simulink model "HIL_model_overall"  (R2014a)
settings: Solver=ode5  StartTime=0.0  StopTime=simulationTime  FixedStep=0.1  RelTol=1e-3
values from neighbouring files (symbols this model uses):
  A_ref = [0.176     0           0 ... (first row only)    [theProgram.m]
  B_ref = [0.0554     0           0 ... (first row only)    [theProgram.m]
  C_ref = [0.05*0.0038     0           0 ... (first row only)    [theProgram.m]
  Di = [50 0 ... (first row only)    [theProgram.m]
  Dist_spv_rfp = sqrt( ( shipL_d(1) - Rfp(1) )^2 + (shipL_d(2) - Rfp(2) )^2 )    [theProgram.m]
  Ds = [-X_u 0 0 ... (first row only)    [theProgram.m]
  iceDiameter = 0.2    [theProgram.m]
  K2_obs = diag([0.25 1 0.5])    [theProgram.m]
  K3_obs = diag([1 1 1])    [theProgram.m]
  K4_obs = diag([250 300 100])    [theProgram.m]
  K_M = [ 1 0 0 ... (first row only)    [theProgram.m]
  K_tow = 20    [theProgram.m]
  kappa = 2    [theProgram.m]
  Kd = [50 0 0 ... (first row only)    [theProgram.m]
  Kp = [10 0 0 ... (first row only)    [theProgram.m]
  Mi_a = iceMass*[1 0; 0 1]    [theProgram.m]
  Mi_rb = iceMass*[1 0; 0 1]    [theProgram.m]
  Ms_a = -[X_udot 0 0 ... (first row only)    [theProgram.m]
  Ms_rb = [shipMass 0 0 ... (first row only)    [theProgram.m]
  Ms_tot = Ms_rb + Ms_a    [theProgram.m]
  Ninstances = 50    [theProgram.m]
  nPoints = size(WP,1)    [theProgram.m]
  Offset_direction = 0    [theProgram.m]
  overturnLimit = 4    [theProgram.m]
  Piceberg = [-4.5; -2.9]    [theProgram.m]
  Pship = [-3.5; -2.9; 0]    [theProgram.m]
  ruptureLimit = 3    [theProgram.m]
  ruptureLimitRef = 9    [theProgram.m]
  ruptureNear = 9.5    [theProgram.m]
  S_trans = [0 -1 0 ... (first row only)    [theProgram.m]
  saved_init = zeros(Ninstances,1)    [theProgram.m]
  sd_break = 0.075*T_break    (= 12)    [theProgram.m]
  sd_overturn = 0.075*T_overturn    (= 9.75)    [theProgram.m]
  sd_slip = 0.075*T_slip    (= 10.5)    [theProgram.m]
  shipL_d = [shipLength-0.55; 0]    [theProgram.m]
  sigma = 0.005    [theProgram.m]
  slippageLimit = 5    [theProgram.m]
  T_bias = diag([20 200 20])    [theProgram.m]
  T_break = 160    [theProgram.m]
  T_overturn = 130    [theProgram.m]
  T_slip = 140    [theProgram.m]
  TowLineLength = 1.11    [theProgram.m]
  u_ref = 0.03    [theProgram.m]
  u_surge_max = 2    [theProgram.m]
  u_sway_max = 1    [theProgram.m]
  u_yaw_max = 2*pi/60    (= 0.10471975512)    [theProgram.m]
  Vc = [cVelocity*cos(cAngle) ... (first row only)    [theProgram.m]
  WP = [-5 -3 ... (first row only)    [theProgram.m]
  WPi_init = 2    [theProgram.m]
libraries: dspmtrx3 x2
(part 1 of 2)
settings Model: Creator=Andreas  LastModifiedBy=mclab
settings DebuggingCC: UnderspecifiedInitializationDetection=Classic  StateNameClashWarn=warning

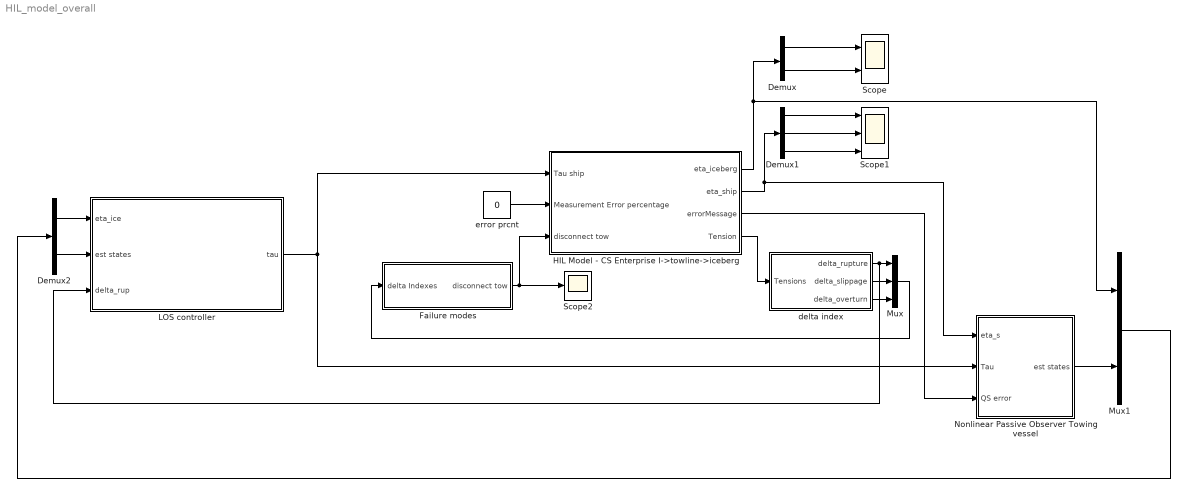
== system HIL_model_overall ==
  Demux : Demux  Outputs=2
  Demux1 : Demux  Outputs=3
  Demux2 : Demux  Outputs=[2; 9]
  Failure modes : Subsystem
  HIL Model - CS Enterprise I->towline->iceberg : Subsystem  VariantControl=Variant1
  LOS controller : Subsystem
  Mux : Mux  Inputs=3
  Mux1 : Mux  Inputs=[2; 9]
  Nonlinear Passive Observer Towing vessel : Subsystem
  Scope : Scope  NumInputPorts=2
      settings: YMin=-5~-5  YMax=5~5  SaveName=ScopeData5
  Scope1 : Scope  NumInputPorts=3
      settings: YMin=-5~-5~-5  YMax=5~5~5  SaveName=ScopeData6
  Scope2 : Scope
      settings: SaveName=ScopeData7
  delta index : Subsystem
  error prcnt : Constant  Value=0
  wires:
  error prcnt/1 -> HIL Model - CS Enterprise I->towline->iceberg/2(Measurement Error percentage)
  HIL Model - CS Enterprise I->towline->iceberg/4(Tension) -> delta index/1(Tensions)
  Failure modes/1(disconnect tow) -> HIL Model - CS Enterprise I->towline->iceberg/3(disconnect tow), Scope2/1
  delta index/2(delta_slippage) -> Mux/2
  delta index/3(delta_overturn) -> Mux/3
  delta index/1(delta_rupture) -> LOS controller/3(delta_rup), Mux/1
  Mux/1 -> Failure modes/1(delta Indexes)
  LOS controller/1(tau) -> HIL Model - CS Enterprise I->towline->iceberg/1(Tau ship), Nonlinear Passive Observer Towing vessel/2(Tau)
  HIL Model - CS Enterprise I->towline->iceberg/1(eta_iceberg) -> Mux1/1, Demux/1
  Demux/2 -> Scope/2
  Demux/1 -> Scope/1
  HIL Model - CS Enterprise I->towline->iceberg/2(eta_ship) -> Nonlinear Passive Observer Towing vessel/1(eta_s), Demux1/1
  Demux1/2 -> Scope1/2
  Demux1/3 -> Scope1/3
  Demux1/1 -> Scope1/1
  HIL Model - CS Enterprise I->towline->iceberg/3(errorMessage) -> Nonlinear Passive Observer Towing vessel/3(QS error)
  Nonlinear Passive Observer Towing vessel/1(est states) -> Mux1/2
  Demux2/2 -> LOS controller/2(est states)
  Demux2/1 -> LOS controller/1(eta_ice)
  Mux1/1 -> Demux2/1

== system HIL_model_overall/Failure modes ==
  delta Indexes : Inport
  Clock : Clock
  MATLAB Function : MATLAB Function  TreatAsAtomicUnit=on
  Memory : Memory
  To Workspace : ToWorkspace  VariableName=isDisconnected  SaveFormat=Timeseries  SampleTime=-1
  limits : Constant  Value=[overturnLimit; ruptureLimit; slippageLimit]  VectorParams1D=off
  disconnect tow : Outport
  wires:
  limits/1 -> MATLAB Function/2(limits)
  delta Indexes/1 -> MATLAB Function/1(deltaIndex)
  Clock/1 -> MATLAB Function/4(theTime)
  MATLAB Function/1(disconnect) -> Memory/1
  Memory/1 -> To Workspace/1, MATLAB Function/3(preDisconnect), disconnect tow/1

== system HIL_model_overall/HIL Model - CS Enterprise I->towline->iceberg ==
  Tau ship : Inport
  Measurement Error percentage : Inport  Port=2
  disconnect tow : Inport  Port=3
  Demux : Demux  Outputs=2
  Mux : Mux  Inputs=[3; 2]
  Ship - Iceberg - Current Model : Subsystem
  Tension estimator : Subsystem
  eta_iceberg : Outport
  eta_ship : Outport  Port=2
  errorMessage : Outport  Port=3
  Tension : Outport  Port=4
  wires:
  Tension estimator/2(T_2dof iceberg) -> Ship - Iceberg - Current Model/2(Tension 2D)
  Tension estimator/1(T_3dof ship) -> Ship - Iceberg - Current Model/1(Tension 3D)
  Measurement Error percentage/1 -> Ship - Iceberg - Current Model/4(error percentage)
  Demux/2 -> Tension estimator/2(eta_i)
  Ship - Iceberg - Current Model/1(eta_i) -> Mux/2, eta_iceberg/1
  Demux/1 -> Tension estimator/1(eta_s)
  Tau ship/1 -> Ship - Iceberg - Current Model/3(tau ship)
  Ship - Iceberg - Current Model/3(error) -> errorMessage/1
  Mux/1 -> Demux/1
  Ship - Iceberg - Current Model/2(eta_s) -> Mux/1, eta_ship/1
  Tension estimator/3(Tension) -> Tension/1
  disconnect tow/1 -> Tension estimator/3(Disconnect towline)

== system HIL_model_overall/LOS controller ==
  eta_ice : Inport
  est states : Inport  Port=2
  delta_rup : Inport  Port=3
  Demux : Demux  Outputs=[3; 3; 3]
  LOS iceberg : Subsystem
  "Point Controller,  backstepping" : Subsystem
  Reference Model : Subsystem
  Waypoints : Constant  Value=WP  VectorParams1D=off
  tau : Outport
  wires:
  eta_ice/1 -> Reference Model/1(eta_ice), LOS iceberg/1(eta_ice)
  Demux/1 -> Reference Model/6(eta_ship est), "Point Controller,  backstepping"/4(eta_s est)
  Demux/2 -> Reference Model/7(nu_ship est), "Point Controller,  backstepping"/5(nu_s est)
  "Point Controller,  backstepping"/1(tau) -> tau/1
  Waypoints/1 -> LOS iceberg/2(WP), Reference Model/5(WP)
  est states/1 -> Demux/1
  Demux/3 -> "Point Controller,  backstepping"/6(b_s est)
  Reference Model/1(eta_d) -> "Point Controller,  backstepping"/1(eta_d)
  Reference Model/2(nu_d) -> "Point Controller,  backstepping"/2(nu_d)
  Reference Model/3(nu_dot_d) -> "Point Controller,  backstepping"/3(nu_dot_d)
  LOS iceberg/1(alpha_iceberg) -> Reference Model/2(alpha_LOS)
  LOS iceberg/2(WPi) -> Reference Model/3(WPi)
  LOS iceberg/3(alphaIce_save) -> Reference Model/4(alpha_LOS_saved)
  delta_rup/1 -> Reference Model/8(delta_rup)

== system HIL_model_overall/Nonlinear Passive Observer Towing vessel ==
  eta_s : Inport
  Tau : Inport  Port=2
  QS error : Inport  Port=3
  Mux : Mux  Inputs=[3; 3; 3]
  To Workspace : ToWorkspace  VariableName=QSerror  SaveFormat=Timeseries  SampleTime=-1
  estimation : Subsystem
  est states : Outport
  wires:
  eta_s/1 -> estimation/1(eta_s)
  estimation/1(eta_s est) -> Mux/1
  Tau/1 -> estimation/2(Tau)
  estimation/2(nu_s est) -> Mux/2
  estimation/3(b_s est) -> Mux/3
  Mux/1 -> est states/1
  QS error/1 -> To Workspace/1, estimation/3(QS error)

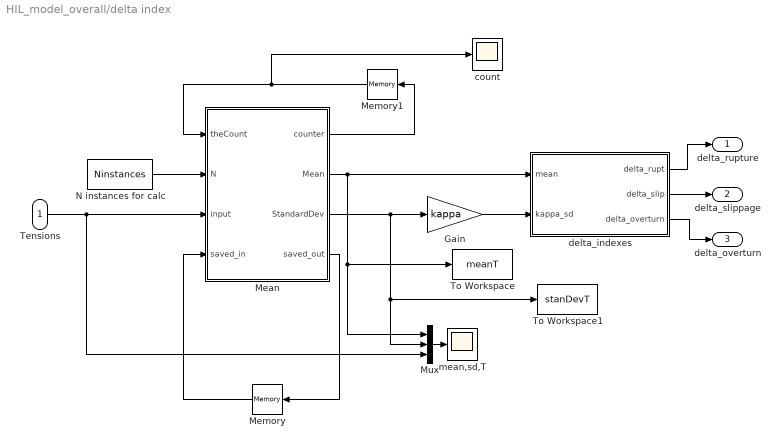
== system HIL_model_overall/delta index ==
  Tensions : Inport
  Gain : Gain  Gain=kappa
  Mean : MATLAB Function  TreatAsAtomicUnit=on
  Memory : Memory  X0=saved_init
  Memory1 : Memory  X0=1
  Mux : Mux  Inputs=3
  N instances for calc : Constant  Value=Ninstances
  To Workspace : ToWorkspace  VariableName=meanT  SaveFormat=Timeseries  SampleTime=-1
  To Workspace1 : ToWorkspace  VariableName=stanDevT  SaveFormat=Timeseries  SampleTime=-1
  count : Scope
  delta_indexes : Subsystem
  mean,sd,T : Scope
      settings: SaveName=ScopeData2
  delta_rupture : Outport
  delta_slippage : Outport  Port=2
  delta_overturn : Outport  Port=3
  wires:
  Mux/1 -> mean,sd,T/1
  Memory/1 -> Mean/4(saved_in)
  Memory1/1 -> Mean/1(theCount), count/1
  Mean/3(StandardDev) -> To Workspace1/1, Mux/2, Gain/1
  Mean/1(counter) -> Memory1/1
  N instances for calc/1 -> Mean/2(N)
  Mean/4(saved_out) -> Memory/1
  Mean/2(Mean) -> To Workspace/1, Mux/1, delta_indexes/1(mean)
  Tensions/1 -> Mux/3, Mean/3(input)
  Gain/1 -> delta_indexes/2(kappa_sd)
  delta_indexes/1(delta_rupt) -> delta_rupture/1
  delta_indexes/2(delta_slip) -> delta_slippage/1
  delta_indexes/3(delta_overturn) -> delta_overturn/1

== system HIL_model_overall/HIL Model - CS Enterprise I->towline->iceberg/Ship - Iceberg - Current Model ==
  Tension 3D : Inport
  Tension 2D : Inport  Port=2
  tau ship : Inport  Port=3
  error percentage : Inport  Port=4
  Current model : Subsystem
  Iceberg model : Subsystem
  MC Lab Signal Fault : MATLAB Function  TreatAsAtomicUnit=on
  Memory : Memory  X0=[0; 0]
  Memory1 : Memory  X0=[0; 0; 0]
  Memory2 : Memory
  Ship model : Subsystem
  eta_i : Outport
  eta_s : Outport  Port=2
  error : Outport  Port=3
  wires:
  Memory2/1 -> MC Lab Signal Fault/4(error_previous)
  Memory1/1 -> MC Lab Signal Fault/5(eta_s_previous)
  Memory/1 -> MC Lab Signal Fault/6(eta_i_previous)
  MC Lab Signal Fault/1(error) -> error/1, Memory2/1
  MC Lab Signal Fault/3(eta_i) -> eta_i/1, Memory/1
  MC Lab Signal Fault/2(eta_s) -> eta_s/1, Memory1/1
  Iceberg model/1(eta_i) -> MC Lab Signal Fault/3(eta_i_in)
  Ship model/2(eta_s) -> MC Lab Signal Fault/2(eta_s_in)
  error percentage/1 -> MC Lab Signal Fault/1(err_percent)
  Ship model/3(nu_s) -> Current model/2(nu_s)  "nu_s"
  Ship model/1(R(psi)^T) -> Current model/1(R(psi) transposed)
  Tension 2D/1 -> Iceberg model/3(T)
  Current model/4(Vc_dot) -> Iceberg model/2(Vc_dot)
  Current model/3(Vc) -> Iceberg model/1(Vc)
  Current model/2(nu_c_dot) -> Ship model/4(nu_c_dot)
  Current model/1(nu_c) -> Ship model/3(nu_c)
  Tension 3D/1 -> Ship model/2(T)
  tau ship/1 -> Ship model/1(Tau)

== system HIL_model_overall/HIL Model - CS Enterprise I->towline->iceberg/Tension estimator ==
  eta_s : Inport
  eta_i : Inport  Port=2
  Disconnect towline : Inport  Port=3
  Constant : Constant  Value=0
  Demux1 : Demux  Outputs=2
  Mux1 : Mux  Inputs=3
  Tension estimate : MATLAB Function  TreatAsAtomicUnit=on
  To Workspace : ToWorkspace  VariableName=tension  SaveFormat=Timeseries  SampleTime=-1
  TowLine Parameters : Constant  Value=[Dist_spv_rfp; TowLineLength; K_tow]  VectorParams1D=off
  T_3dof ship : Outport
  T_2dof iceberg : Outport  Port=2
  Tension : Outport  Port=3
  wires:
  Tension estimate/1(Tension) -> T_2dof iceberg/1, Demux1/1
  TowLine Parameters/1 -> Tension estimate/3(TowLineParameters)
  Constant/1 -> Mux1/3
  Demux1/2 -> Mux1/2
  Demux1/1 -> Mux1/1
  Mux1/1 -> T_3dof ship/1
  eta_s/1 -> Tension estimate/1(eta_s_in)
  eta_i/1 -> Tension estimate/2(eta_i_in)
  Tension estimate/2(T) -> To Workspace/1, Tension/1
  Disconnect towline/1 -> Tension estimate/4(disconnected)

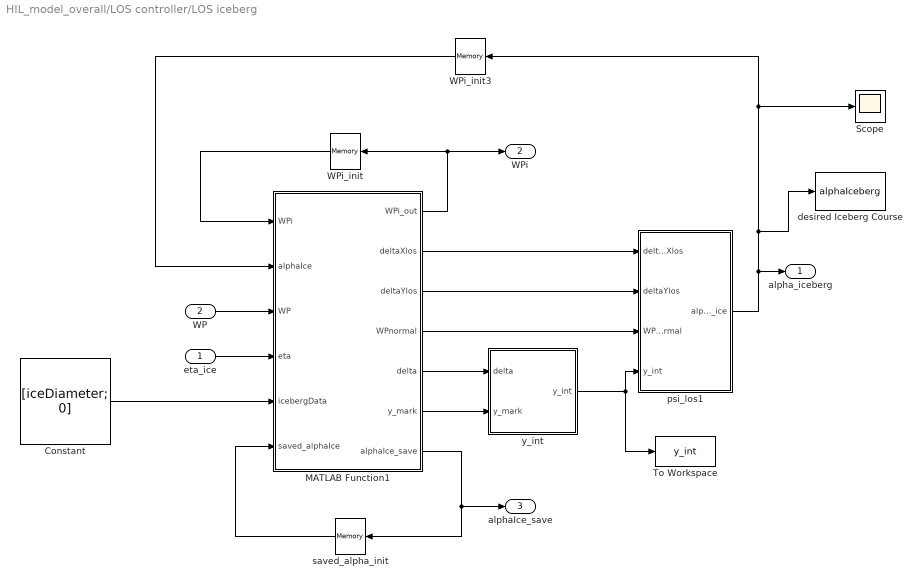
== system HIL_model_overall/LOS controller/LOS iceberg ==
  eta_ice : Inport
  WP : Inport  Port=2
  Constant : Constant  Value=[iceDiameter; 0]  VectorParams1D=off
  MATLAB Function1 : MATLAB Function  TreatAsAtomicUnit=on
  Scope : Scope
      settings: SaveName=ScopeData2
  To Workspace : ToWorkspace  VariableName=y_int  SaveFormat=Timeseries  SampleTime=-1
  WPi_init : Memory  X0=WPi_init  InheritSampleTime=on
  WPi_init3 : Memory  InheritSampleTime=on
  desired Iceberg Course : ToWorkspace  VariableName=alphaIceberg  SaveFormat=Timeseries  SampleTime=-1
  psi_los1 : Subsystem
  saved_alpha_init : Memory  InheritSampleTime=on
  y_int : Subsystem
  alpha_iceberg : Outport
  WPi : Outport  Port=2
  alphaIce_save : Outport  Port=3
  wires:
  eta_ice/1 -> MATLAB Function1/4(eta)
  WP/1 -> MATLAB Function1/3(WP)
  MATLAB Function1/1(WPi_out) -> WPi_init/1, WPi/1
  WPi_init/1 -> MATLAB Function1/1(WPi)
  MATLAB Function1/2(deltaXlos) -> psi_los1/1(deltaXlos)
  MATLAB Function1/3(deltaYlos) -> psi_los1/2(deltaYlos)
  y_int/1(y_int) -> To Workspace/1, psi_los1/4(y_int)
  psi_los1/1(alpha_ice) -> desired Iceberg Course/1, Scope/1, WPi_init3/1, alpha_iceberg/1
  MATLAB Function1/6(y_mark) -> y_int/2(y_mark)
  MATLAB Function1/5(delta) -> y_int/1(delta)
  MATLAB Function1/4(WPnormal) -> psi_los1/3(WPnormal)
  Constant/1 -> MATLAB Function1/5(icebergData)
  MATLAB Function1/7(alphaIce_save) -> saved_alpha_init/1, alphaIce_save/1
  saved_alpha_init/1 -> MATLAB Function1/6(saved_alphaIce)
  WPi_init3/1 -> MATLAB Function1/2(alphaIce)

== system HIL_model_overall/LOS controller/Point Controller,  backstepping ==
  eta_d : Inport
  nu_d : Inport  Port=2
  nu_dot_d : Inport  Port=3
  eta_s est : Inport  Port=4
  nu_s est : Inport  Port=5
  b_s est : Inport  Port=6
  Demux : Demux  Outputs=3
  Scope : Scope  NumInputPorts=3
      settings: TimeRange=400  YMin=0.776~0.0235~-0.00225  YMax=0.777~0.028~-0.00195  SaveName=ScopeData5  MaxDataPoints=10000
  Tau : Subsystem
  alpha1_dot : Subsystem
  alpha_1 : Subsystem
  z1 : Subsystem
  z2 : Subsystem
  tau : Outport
  wires:
  Tau/1(tau) -> tau/1, Demux/1
  Demux/2 -> Scope/2
  Demux/3 -> Scope/3
  Demux/1 -> Scope/1
  b_s est/1 -> Tau/6(b_s est)
  alpha1_dot/5(alpha_1_dot) -> Tau/5(alpha1_dot)
  eta_d/1 -> z1/1(eta_d)
  eta_s est/1 -> z1/2(eta_ship)
  z1/1(z1) -> alpha_1/1(z1)
  z1/3(eta des) -> alpha_1/3(eta_d)
  z1/2(eta_s) -> alpha_1/2(eta_s)
  nu_d/1 -> alpha_1/4(nu_d)
  nu_s est/1 -> alpha1_dot/6(nu_s), z2/6(nu_ship)
  alpha_1/1(alpha_1) -> z2/1(alpha_1)
  alpha_1/2(z 1) -> z2/2(z1)
  alpha_1/5(eta d) -> z2/5(eta_d)
  alpha_1/3(nu d) -> z2/3(nu_d)
  alpha_1/4(eta s) -> z2/4(eta_s)
  nu_dot_d/1 -> alpha1_dot/7(nu_dot_d)
  z2/1(z2) -> alpha1_dot/1(z2)
  z2/4(eta s) -> alpha1_dot/4(eta_s)
  z2/5(eta d) -> alpha1_dot/5(eta_d)
  z2/2(z 1) -> alpha1_dot/2(z1)
  z2/3(nu d) -> alpha1_dot/3(nu_d)
  alpha1_dot/1(z 1) -> Tau/1(z1)
  alpha1_dot/2(z 2) -> Tau/2(z2)
  alpha1_dot/3(nu s) -> Tau/3(nu_s)
  alpha1_dot/4(eta s) -> Tau/4(eta_s)

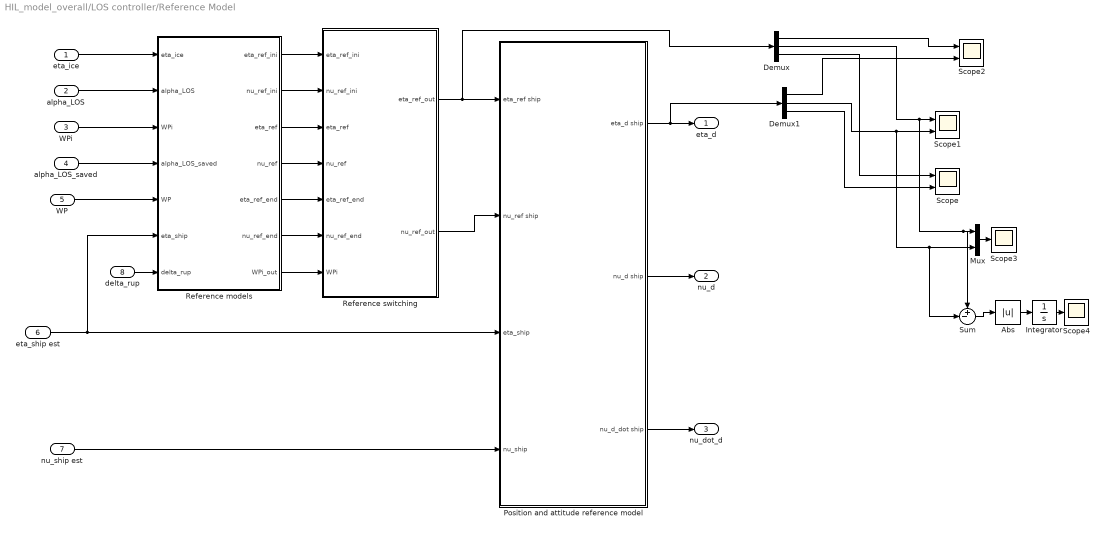
== system HIL_model_overall/LOS controller/Reference Model ==
  eta_ice : Inport
  alpha_LOS : Inport  Port=2
  WPi : Inport  Port=3
  alpha_LOS_saved : Inport  Port=4
  WP : Inport  Port=5
  eta_ship est : Inport  Port=6
  nu_ship est : Inport  Port=7
  delta_rup : Inport  Port=8
  Abs : Abs
  Demux : Demux  Outputs=3
  Demux1 : Demux  Outputs=3
  Integrator : Integrator
  Mux : Mux  Inputs=2
  Position and attitude reference model : Subsystem
  Reference models : Subsystem
  Reference switching : Subsystem
  Scope : Scope  NumInputPorts=2
      settings: TimeRange=500  YMin=-5~-5  YMax=5~5  SaveName=ScopeData9
  Scope1 : Scope  NumInputPorts=2
      settings: TimeRange=500  YMin=-5~-5  YMax=5~5  SaveName=ScopeData11
  Scope2 : Scope  NumInputPorts=2
      settings: TimeRange=500  YMin=-5~-5  YMax=5~5  SaveName=ScopeData12
  Scope3 : Scope
      settings: SaveName=ScopeData16
  Scope4 : Scope
      settings: SaveName=ScopeData17
  Sum : Sum  Inputs=+-|
  eta_d : Outport
  nu_d : Outport  Port=2
  nu_dot_d : Outport  Port=3
  wires:
  Position and attitude reference model/1(eta_d ship) -> Demux1/1, eta_d/1
  Position and attitude reference model/2(nu_d ship) -> nu_d/1
  Position and attitude reference model/3(nu_d_dot ship) -> nu_dot_d/1
  eta_ice/1 -> Reference models/1(eta_ice)
  Reference models/6(nu_ref_end) -> Reference switching/6(nu_ref_end)
  Reference models/1(eta_ref_ini) -> Reference switching/1(eta_ref_ini)
  alpha_LOS_saved/1 -> Reference models/4(alpha_LOS_saved)
  Reference models/4(nu_ref) -> Reference switching/4(nu_ref)
  eta_ship est/1 -> Position and attitude reference model/3(eta_ship), Reference models/6(eta_ship)
  WP/1 -> Reference models/5(WP)
  Reference models/7(WPi_out) -> Reference switching/7(WPi)
  Reference switching/2(nu_ref_out) -> Position and attitude reference model/2(nu_ref ship)
  Reference models/2(nu_ref_ini) -> Reference switching/2(nu_ref_ini)
  Reference models/3(eta_ref) -> Reference switching/3(eta_ref)
  Reference models/5(eta_ref_end) -> Reference switching/5(eta_ref_end)
  WPi/1 -> Reference models/3(WPi)
  alpha_LOS/1 -> Reference models/2(alpha_LOS)
  nu_ship est/1 -> Position and attitude reference model/4(nu_ship)
  Reference switching/1(eta_ref_out) -> Demux/1, Position and attitude reference model/1(eta_ref ship)
  Demux1/3 -> Scope/2
  Demux/3 -> Scope/1
  Demux/2 -> Sum/1, Mux/1, Scope1/1
  Demux1/2 -> Sum/2, Mux/2, Scope1/2
  Demux/1 -> Scope2/1
  Demux1/1 -> Scope2/2
  Mux/1 -> Scope3/1
  Sum/1 -> Abs/1
  Abs/1 -> Integrator/1
  Integrator/1 -> Scope4/1
  delta_rup/1 -> Reference models/7(delta_rup)

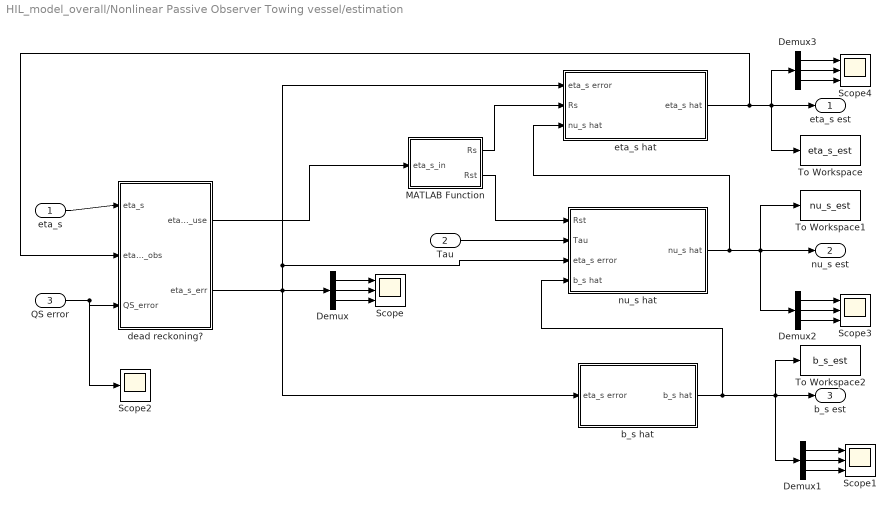
== system HIL_model_overall/Nonlinear Passive Observer Towing vessel/estimation ==
  eta_s : Inport
  Tau : Inport  Port=2
  QS error : Inport  Port=3
  Demux{,1..3} (4 alike) : Demux  Outputs=3
  MATLAB Function : MATLAB Function  TreatAsAtomicUnit=on
  Scope{,1,3..4} (4 alike) : Scope  NumInputPorts=3
      Scope settings: YMin=-5~-5~-5  YMax=5~5~5
      Scope1 settings: YMin=-5~-5~-5  YMax=5~5~5  SaveName=ScopeData15
      Scope3 settings: YMin=-5~-5~-5  YMax=5~5~5  SaveName=ScopeData3
      Scope4 settings: YMin=-5~-5~-5  YMax=5~5~5  SaveName=ScopeData8
  Scope2 : Scope
      settings: SaveName=ScopeData23
  To Workspace : ToWorkspace  VariableName=eta_s_est  SaveFormat=Timeseries  SampleTime=-1
  To Workspace1 : ToWorkspace  VariableName=nu_s_est  SaveFormat=Timeseries  SampleTime=-1
  To Workspace2 : ToWorkspace  VariableName=b_s_est  SaveFormat=Timeseries  SampleTime=-1
  b_s hat : Subsystem
  dead reckoning? : MATLAB Function  TreatAsAtomicUnit=on
  eta_s hat : Subsystem
  nu_s hat : Subsystem
  eta_s est : Outport
  nu_s est : Outport  Port=2
  b_s est : Outport  Port=3
  wires:
  MATLAB Function/1(Rs) -> eta_s hat/2(Rs)
  eta_s hat/1(eta_s hat) -> dead reckoning?/2(eta_s_obs), Demux3/1, To Workspace/1, eta_s est/1
  nu_s hat/1(nu_s hat) -> To Workspace1/1, Demux2/1, nu_s est/1, eta_s hat/3(nu_s hat)
  MATLAB Function/2(Rst) -> nu_s hat/1(Rst)
  Tau/1 -> nu_s hat/2(Tau)
  b_s hat/1(b_s hat) -> To Workspace2/1, Demux1/1, b_s est/1, nu_s hat/4(b_s hat)
  Demux/1 -> Scope/1
  Demux/2 -> Scope/2
  Demux/3 -> Scope/3
  Demux1/1 -> Scope1/1
  Demux1/2 -> Scope1/2
  Demux1/3 -> Scope1/3
  eta_s/1 -> dead reckoning?/1(eta_s)
  QS error/1 -> dead reckoning?/3(QS_error), Scope2/1
  dead reckoning?/1(eta_s_use) -> MATLAB Function/1(eta_s_in)
  dead reckoning?/2(eta_s_err) -> b_s hat/1(eta_s error), nu_s hat/3(eta_s error), eta_s hat/1(eta_s error), Demux/1
  Demux2/1 -> Scope3/1
  Demux2/2 -> Scope3/2
  Demux2/3 -> Scope3/3
  Demux3/1 -> Scope4/1
  Demux3/2 -> Scope4/2
  Demux3/3 -> Scope4/3

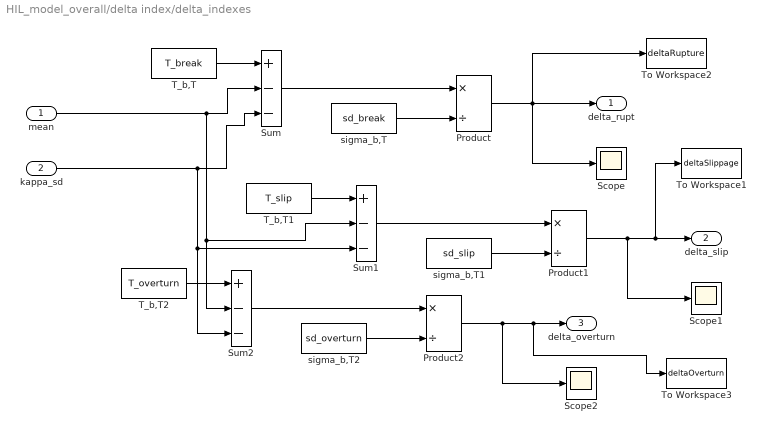
== system HIL_model_overall/delta index/delta_indexes ==
  mean : Inport
  kappa_sd : Inport  Port=2
  Product : Product  Inputs=*/
  Product1 : Product  Inputs=*/
  Product2 : Product  Inputs=*/
  Scope : Scope
  Scope1 : Scope
      settings: SaveName=ScopeData3
  Scope2 : Scope
      settings: SaveName=ScopeData4
  Sum : Sum  Inputs=+--
  Sum1 : Sum  Inputs=+--
  Sum2 : Sum  Inputs=+--
  T_b,T : Constant  Value=T_break
  T_b,T1 : Constant  Value=T_slip
  T_b,T2 : Constant  Value=T_overturn
  To Workspace1 : ToWorkspace  VariableName=deltaSlippage  SaveFormat=Timeseries  SampleTime=-1
  To Workspace2 : ToWorkspace  VariableName=deltaRupture  SaveFormat=Timeseries  SampleTime=-1
  To Workspace3 : ToWorkspace  VariableName=deltaOverturn  SaveFormat=Timeseries  SampleTime=-1
  sigma_b,T : Constant  Value=sd_break
  sigma_b,T1 : Constant  Value=sd_slip
  sigma_b,T2 : Constant  Value=sd_overturn
  delta_rupt : Outport
  delta_slip : Outport  Port=2
  delta_overturn : Outport  Port=3
  wires:
  Product/1 -> To Workspace2/1, delta_rupt/1, Scope/1
  kappa_sd/1 -> Sum2/3, Sum1/3, Sum/3
  sigma_b,T/1 -> Product/2
  Sum/1 -> Product/1
  T_b,T/1 -> Sum/1
  mean/1 -> Sum2/2, Sum1/2, Sum/2
  Product1/1 -> To Workspace1/1, delta_slip/1, Scope1/1
  sigma_b,T1/1 -> Product1/2
  Sum1/1 -> Product1/1
  T_b,T1/1 -> Sum1/1
  Product2/1 -> To Workspace3/1, delta_overturn/1, Scope2/1
  sigma_b,T2/1 -> Product2/2
  Sum2/1 -> Product2/1
  T_b,T2/1 -> Sum2/1

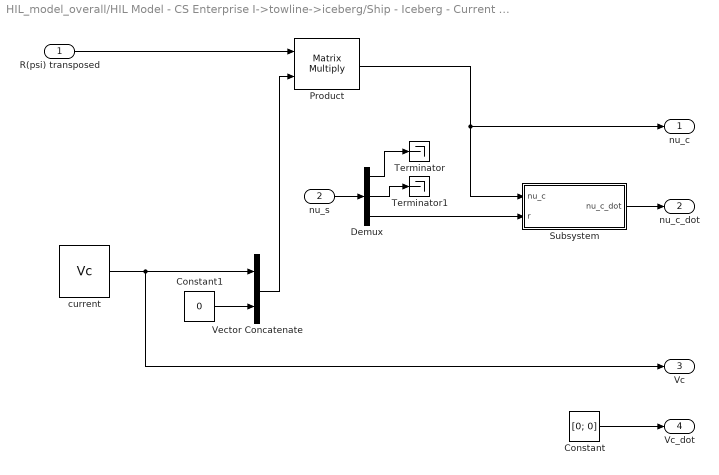
== system HIL_model_overall/HIL Model - CS Enterprise I->towline->iceberg/Ship - Iceberg - Current Model/Current model ==
  R(psi) transposed : Inport
  nu_s : Inport  Port=2
  Constant : Constant  Value=[0; 0]  VectorParams1D=off
  Constant1 : Constant  Value=0
  Demux : Demux  Outputs=3
  Product : Product  Multiplication=Matrix(*)
  Subsystem : Subsystem
  Terminator : Terminator
  Terminator1 : Terminator
  Vector Concatenate : Concatenate  Mode=Multidimensional array
  current : Constant  Value=Vc  VectorParams1D=off
  nu_c : Outport
  nu_c_dot : Outport  Port=2
  Vc : Outport  Port=3
  Vc_dot : Outport  Port=4
  wires:
  Vector Concatenate/1 -> Product/2
  Constant1/1 -> Vector Concatenate/2
  Constant/1 -> Vc_dot/1
  Subsystem/1(nu_c_dot) -> nu_c_dot/1
  Demux/3 -> Subsystem/2(r)
  Demux/2 -> Terminator1/1
  Demux/1 -> Terminator/1
  nu_s/1 -> Demux/1
  Product/1 -> nu_c/1, Subsystem/1(nu_c)
  R(psi) transposed/1 -> Product/1
  current/1 -> Vector Concatenate/1, Vc/1

== system HIL_model_overall/HIL Model - CS Enterprise I->towline->iceberg/Ship - Iceberg - Current Model/Iceberg model ==
  Vc : Inport
  Vc_dot : Inport  Port=2
  T : Inport  Port=3
  Demux1 : Demux  Outputs=2
  Di : Gain  Gain=Di  Multiplication=Matrix(K*u) (u vector)
  Integrator1 : Integrator  InitialCondition=Piceberg
  Integrator3 : Integrator  InitialCondition=[0;0]
  M-1 i : Gain  Gain=inv(Mi_rb + Mi_a)  Multiplication=Matrix(K*u)
  Mi_a : Gain  Gain=Mi_a  Multiplication=Matrix(K*u) (u vector)
  Subtract1 : Sum  Inputs=++-
  Sum : Sum  Inputs=|-+
  To Workspace3 : ToWorkspace  VariableName=x_i  SaveFormat=Timeseries  SampleTime=-1
  To Workspace4 : ToWorkspace  VariableName=y_i  SaveFormat=Timeseries  SampleTime=-1
  nu_i : ToWorkspace  VariableName=nu_i  SaveFormat=Timeseries  SampleTime=-1
  eta_i : Outport
  wires:
  Demux1/2 -> To Workspace4/1
  Demux1/1 -> To Workspace3/1
  Di/1 -> Subtract1/3
  Sum/1 -> Di/1
  Vc/1 -> Sum/1
  Mi_a/1 -> Subtract1/2
  Vc_dot/1 -> Mi_a/1
  T/1 -> Subtract1/1
  Subtract1/1 -> M-1 i/1
  M-1 i/1 -> Integrator3/1
  Integrator1/1 -> eta_i/1, Demux1/1  "eta_i"
  Integrator3/1 -> Integrator1/1, nu_i/1, Sum/2  "nu_i"

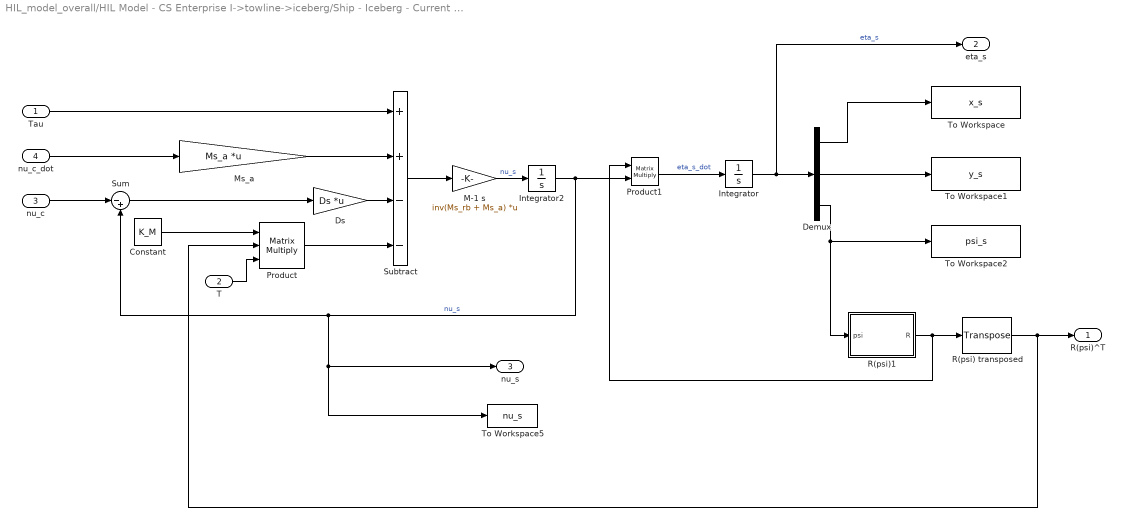
== system HIL_model_overall/HIL Model - CS Enterprise I->towline->iceberg/Ship - Iceberg - Current Model/Ship model ==
  Tau : Inport
  T : Inport  Port=2
  nu_c : Inport  Port=3
  nu_c_dot : Inport  Port=4
  Constant : Constant  Value=K_M  VectorParams1D=off
  Demux : Demux  Outputs=3
  Ds : Gain  Gain=Ds  Multiplication=Matrix(K*u) (u vector)
  Integrator : Integrator  InitialCondition=Pship
  Integrator2 : Integrator  InitialCondition=[0; 0; 0]
  M-1 s : Gain  Gain=inv(Ms_rb + Ms_a)  Multiplication=Matrix(K*u) (u vector)
  Ms_a : Gain  Gain=Ms_a  Multiplication=Matrix(K*u) (u vector)
  Product : Product  Inputs=***  Multiplication=Matrix(*)
  Product1 : Product  Multiplication=Matrix(*)
  R(psi) transposed : dspmtrx3/Transpose  Hermitian=off  overflowFlag=off
  R(psi)1 : MATLAB Function  TreatAsAtomicUnit=on
  Subtract : Sum  Inputs=++--
  Sum : Sum  Inputs=|-+
  To Workspace : ToWorkspace  VariableName=x_s  SaveFormat=Timeseries  SampleTime=-1
  To Workspace1 : ToWorkspace  VariableName=y_s  SaveFormat=Timeseries  SampleTime=-1
  To Workspace2 : ToWorkspace  VariableName=psi_s  SaveFormat=Timeseries  SampleTime=-1
  To Workspace5 : ToWorkspace  VariableName=nu_s  SaveFormat=Timeseries  SampleTime=-1
  R(psi)^T : Outport
  eta_s : Outport  Port=2
  nu_s : Outport  Port=3
  wires:
  Tau/1 -> Subtract/1
  R(psi) transposed/1 -> R(psi)^T/1, Product/2
  Demux/3 -> To Workspace2/1, R(psi)1/1(psi)
  Demux/2 -> To Workspace1/1
  Demux/1 -> To Workspace/1
  Product1/1 -> Integrator/1  "eta_s_dot"
  R(psi)1/1(R) -> R(psi) transposed/1, Product1/1
  Constant/1 -> Product/1
  Subtract/1 -> M-1 s/1
  M-1 s/1 -> Integrator2/1  "nu_s"
  Ds/1 -> Subtract/3
  Ms_a/1 -> Subtract/2
  Integrator/1 -> Demux/1, eta_s/1  "eta_s"
  T/1 -> Product/3
  nu_c/1 -> Sum/1
  Sum/1 -> Ds/1
  Integrator2/1 -> nu_s/1, To Workspace5/1, Sum/2, Product1/2  "nu_s"
  Product/1 -> Subtract/4
  nu_c_dot/1 -> Ms_a/1

== system HIL_model_overall/LOS controller/LOS iceberg/psi_los1 ==
  deltaXlos : Inport
  deltaYlos : Inport  Port=2
  WPnormal : Inport  Port=3
  y_int : Inport  Port=4
  Gain : Gain  Gain=sigma
  Sum : Sum  Inputs=|++
  Sum1 : Sum  Inputs=|++
  Trigonometric Function : Trigonometry  Operator=atan2
  c : Trigonometry  Operator=cos
  s : Trigonometry
  y_int x : Product
  y_int y : Product
  alpha_ice : Outport
  wires:
  Trigonometric Function/1 -> alpha_ice/1
  Sum1/1 -> Trigonometric Function/1
  Sum/1 -> Trigonometric Function/2
  deltaYlos/1 -> Sum1/1
  deltaXlos/1 -> Sum/1
  c/1 -> y_int x/2
  s/1 -> y_int y/2
  Gain/1 -> y_int y/1, y_int x/1
  y_int/1 -> Gain/1
  WPnormal/1 -> c/1, s/1
  y_int x/1 -> Sum/2
  y_int y/1 -> Sum1/2

== system HIL_model_overall/LOS controller/LOS iceberg/y_int ==
  delta : Inport
  y_mark : Inport  Port=2
  Divide : Product  Inputs=*/
  Gain : Gain  Gain=sigma
  Integrator2 : Integrator
  Scope1 : Scope
      settings: SaveName=ScopeData4
  Sum : Sum  Inputs=|++
  Sum1 : Sum  Inputs=|++
  WPi_init2 : Memory  InheritSampleTime=on
  delta*delta : Product
  delta*y : Product
  square : Product
  y_int : Outport
  wires:
  delta/1 -> delta*delta/2, delta*delta/1, delta*y/1
  y_mark/1 -> Sum/1, delta*y/2
  WPi_init2/1 -> Gain/1
  Gain/1 -> Sum/2
  Sum/1 -> square/2, square/1
  square/1 -> Sum1/2
  delta*delta/1 -> Sum1/1
  delta*y/1 -> Divide/1
  Sum1/1 -> Divide/2
  Divide/1 -> Integrator2/1
  Integrator2/1 -> WPi_init2/1, Scope1/1, y_int/1

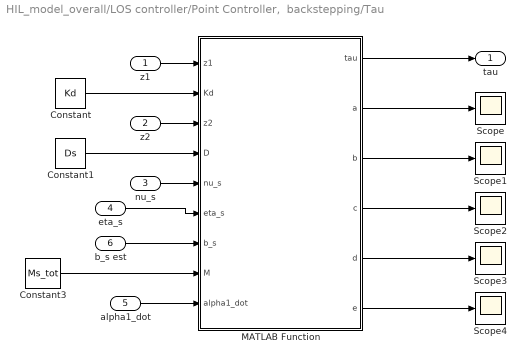
== system HIL_model_overall/LOS controller/Point Controller,  backstepping/Tau ==
  z1 : Inport
  z2 : Inport  Port=2
  nu_s : Inport  Port=3
  eta_s : Inport  Port=4
  alpha1_dot : Inport  Port=5
  b_s est : Inport  Port=6
  Constant : Constant  Value=Kd  VectorParams1D=off
  Constant1 : Constant  Value=Ds  VectorParams1D=off
  Constant3 : Constant  Value=Ms_tot  VectorParams1D=off
  MATLAB Function : MATLAB Function  TreatAsAtomicUnit=on
  Scope{,1..4} (5 alike) : Scope
      Scope settings: SaveName=ScopeData6
      Scope1 settings: YMin=-0.02  YMax=0.1  SaveName=ScopeData7
      Scope2 settings: SaveName=ScopeData10
      Scope3 settings: SaveName=ScopeData13
      Scope4 settings: SaveName=ScopeData14
  tau : Outport
  wires:
  Constant/1 -> MATLAB Function/2(Kd)
  MATLAB Function/1(tau) -> tau/1
  z2/1 -> MATLAB Function/3(z2)
  z1/1 -> MATLAB Function/1(z1)
  Constant1/1 -> MATLAB Function/4(D)
  nu_s/1 -> MATLAB Function/5(nu_s)
  eta_s/1 -> MATLAB Function/6(eta_s)
  Constant3/1 -> MATLAB Function/8(M)
  alpha1_dot/1 -> MATLAB Function/9(alpha1_dot)
  MATLAB Function/2(a) -> Scope/1
  MATLAB Function/3(b) -> Scope1/1
  MATLAB Function/4(c) -> Scope2/1
  MATLAB Function/5(d) -> Scope3/1
  MATLAB Function/6(e) -> Scope4/1
  b_s est/1 -> MATLAB Function/7(b_s)

== system HIL_model_overall/LOS controller/Point Controller,  backstepping/alpha1_dot ==
  z2 : Inport
  z1 : Inport  Port=2
  nu_d : Inport  Port=3
  eta_s : Inport  Port=4
  eta_d : Inport  Port=5
  nu_s : Inport  Port=6
  nu_dot_d : Inport  Port=7
  Constant : Constant  Value=Kp  VectorParams1D=off
  Constant1 : Constant  Value=S_trans  VectorParams1D=off
  MATLAB Function : MATLAB Function  TreatAsAtomicUnit=on
  z 1 : Outport
  z 2 : Outport  Port=2
  nu s : Outport  Port=3
  eta s : Outport  Port=4
  alpha_1_dot : Outport  Port=5
  wires:
  z1/1 -> z 1/1, MATLAB Function/3(z1)
  Constant/1 -> MATLAB Function/1(Kp)
  MATLAB Function/1(alpha_1_dot) -> alpha_1_dot/1
  z2/1 -> z 2/1, MATLAB Function/2(z2)
  Constant1/1 -> MATLAB Function/5(S)
  eta_s/1 -> eta s/1, MATLAB Function/6(eta_s)
  nu_s/1 -> nu s/1, MATLAB Function/4(nu_s)
  nu_d/1 -> MATLAB Function/8(nu_d)
  nu_dot_d/1 -> MATLAB Function/9(nu_dot_d)
  eta_d/1 -> MATLAB Function/7(eta_d)

== system HIL_model_overall/LOS controller/Point Controller,  backstepping/alpha_1 ==
  z1 : Inport
  eta_s : Inport  Port=2
  eta_d : Inport  Port=3
  nu_d : Inport  Port=4
  Constant : Constant  Value=Kp  VectorParams1D=off
  MATLAB Function : MATLAB Function  TreatAsAtomicUnit=on
  alpha_1 : Outport
  z 1 : Outport  Port=2
  nu d : Outport  Port=3
  eta s : Outport  Port=4
  eta d : Outport  Port=5
  wires:
  z1/1 -> z 1/1, MATLAB Function/2(z1)
  Constant/1 -> MATLAB Function/1(Kp)
  MATLAB Function/1(alpha_1) -> alpha_1/1
  nu_d/1 -> nu d/1, MATLAB Function/3(nu_d)
  eta_d/1 -> eta d/1, MATLAB Function/5(eta_d)
  eta_s/1 -> eta s/1, MATLAB Function/4(eta_s)

== system HIL_model_overall/LOS controller/Point Controller,  backstepping/z1 ==
  eta_d : Inport
  eta_ship : Inport  Port=2
  Product : Product  Multiplication=Matrix(*)
  R(psi) transposed : dspmtrx3/Transpose  Hermitian=off  overflowFlag=off
  R(psi)1 : MATLAB Function  TreatAsAtomicUnit=on
  Scope1 : Scope  NumInputPorts=2
      settings: YMin=-5~-5  YMax=5~5  SaveName=ScopeData20
  Sum : Sum  Inputs=|+-
  z1 : Outport
  eta_s : Outport  Port=2
  eta des : Outport  Port=3
  wires:
  eta_ship/1 -> eta_s/1, Scope1/1, Sum/1, R(psi)1/1(eta)
  R(psi)1/1(R) -> R(psi) transposed/1
  R(psi) transposed/1 -> Product/1
  eta_d/1 -> Scope1/2, eta des/1, Sum/2
  Sum/1 -> Product/2
  Product/1 -> z1/1

== system HIL_model_overall/LOS controller/Point Controller,  backstepping/z2 ==
  alpha_1 : Inport
  z1 : Inport  Port=2
  nu_d : Inport  Port=3
  eta_s : Inport  Port=4
  eta_d : Inport  Port=5
  nu_ship : Inport  Port=6
  MATLAB Function : MATLAB Function  TreatAsAtomicUnit=on
  z2 : Outport
  z 1 : Outport  Port=2
  nu d : Outport  Port=3
  eta s : Outport  Port=4
  eta d : Outport  Port=5
  wires:
  nu_ship/1 -> MATLAB Function/1(nu_ship)
  alpha_1/1 -> MATLAB Function/2(alpha1)
  MATLAB Function/1(z2) -> z2/1
  z1/1 -> z 1/1
  nu_d/1 -> nu d/1
  eta_s/1 -> eta s/1
  eta_d/1 -> eta d/1

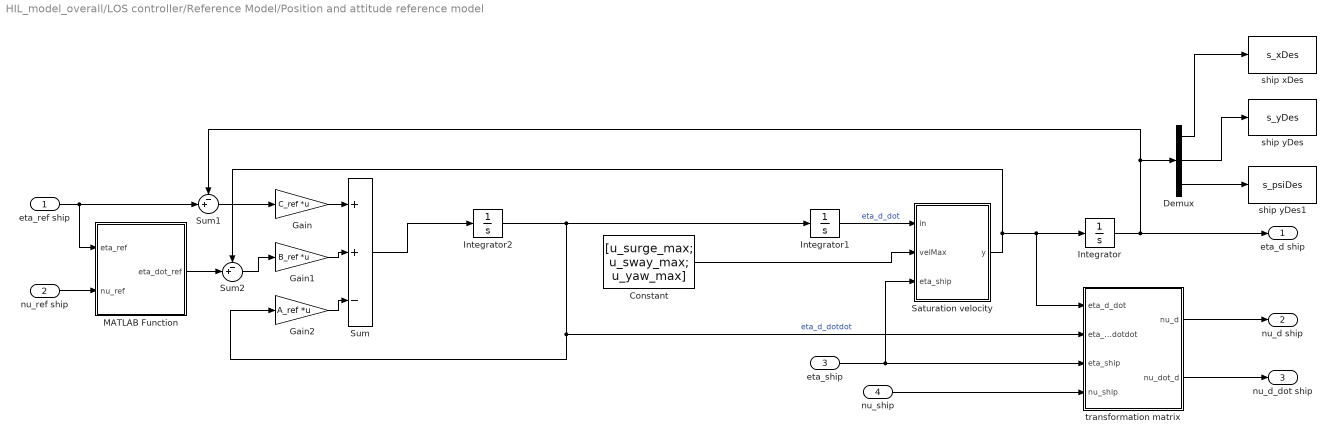
== system HIL_model_overall/LOS controller/Reference Model/Position and attitude reference model ==
  eta_ref ship : Inport
  nu_ref ship : Inport  Port=2
  eta_ship : Inport  Port=3
  nu_ship : Inport  Port=4
  Constant : Constant  Value=[u_surge_max; u_sway_max; u_yaw_max]  VectorParams1D=off
  Demux : Demux  Outputs=3
  Gain : Gain  Gain=C_ref  Multiplication=Matrix(K*u)
  Gain1 : Gain  Gain=B_ref  Multiplication=Matrix(K*u)
  Gain2 : Gain  Gain=A_ref  Multiplication=Matrix(K*u)
  Integrator : Integrator  InitialCondition=Pship
  Integrator1 : Integrator  InitialCondition=[0;0;0]
  Integrator2 : Integrator  InitialCondition=[0;0;0]
  MATLAB Function : MATLAB Function  TreatAsAtomicUnit=on
  Saturation velocity : MATLAB Function  TreatAsAtomicUnit=on
  Sum : Sum  Inputs=++-
  Sum1 : Sum  Inputs=-+|
  Sum2 : Sum  Inputs=-+|
  ship xDes : ToWorkspace  VariableName=s_xDes  SaveFormat=Timeseries  SampleTime=-1
  ship yDes : ToWorkspace  VariableName=s_yDes  SaveFormat=Timeseries  SampleTime=-1
  ship yDes1 : ToWorkspace  VariableName=s_psiDes  SaveFormat=Timeseries  SampleTime=-1
  transformation matrix : MATLAB Function  TreatAsAtomicUnit=on
  eta_d ship : Outport
  nu_d ship : Outport  Port=2
  nu_d_dot ship : Outport  Port=3
  wires:
  Gain/1 -> Sum/1
  Sum1/1 -> Gain/1
  eta_ref ship/1 -> MATLAB Function/1(eta_ref), Sum1/2
  Saturation velocity/1(y) -> Integrator/1, transformation matrix/1(eta_d_dot), Sum2/1
  Constant/1 -> Saturation velocity/2(velMax)
  eta_ship/1 -> Saturation velocity/3(eta_ship), transformation matrix/3(eta_ship)
  Integrator1/1 -> Saturation velocity/1(in)  "eta_d_dot"
  Gain1/1 -> Sum/2
  Gain2/1 -> Sum/3
  Sum/1 -> Integrator2/1
  transformation matrix/2(nu_dot_d) -> nu_d_dot ship/1
  nu_ship/1 -> transformation matrix/4(nu_ship)
  Demux/2 -> ship yDes/1
  Demux/1 -> ship xDes/1
  Integrator2/1 -> Gain2/1, transformation matrix/2(eta_d_dotdot), Integrator1/1  "eta_d_dotdot"
  nu_ref ship/1 -> MATLAB Function/2(nu_ref)
  Sum2/1 -> Gain1/1
  MATLAB Function/1(eta_dot_ref) -> Sum2/2
  transformation matrix/1(nu_d) -> nu_d ship/1
  Integrator/1 -> eta_d ship/1, Sum1/1, Demux/1
  Demux/3 -> ship yDes1/1

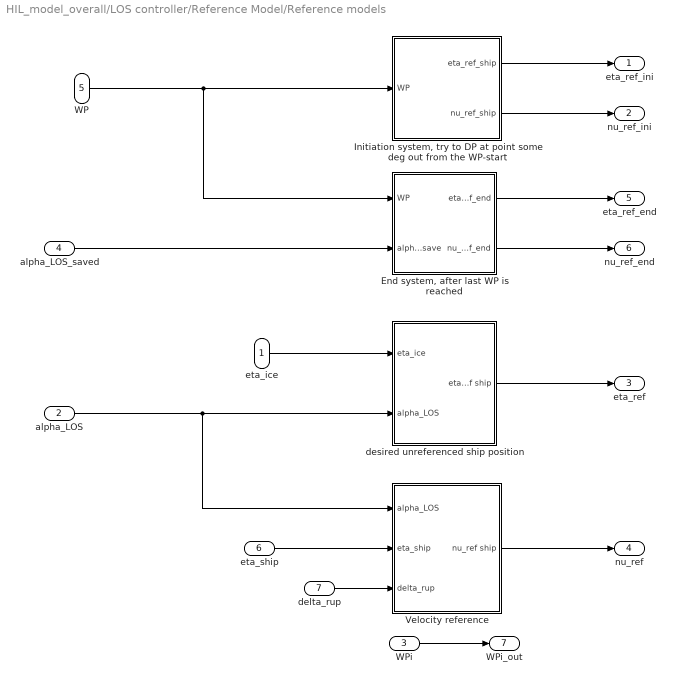
== system HIL_model_overall/LOS controller/Reference Model/Reference models ==
  eta_ice : Inport
  alpha_LOS : Inport  Port=2
  WPi : Inport  Port=3
  alpha_LOS_saved : Inport  Port=4
  WP : Inport  Port=5
  eta_ship : Inport  Port=6
  delta_rup : Inport  Port=7
  "End system, after last WP is reached " : Subsystem
  "Initiation system, try to DP at point some deg out from the WP-start" : Subsystem
  Velocity reference : Subsystem
  desired unreferenced ship position : Subsystem
  eta_ref_ini : Outport
  nu_ref_ini : Outport  Port=2
  eta_ref : Outport  Port=3
  nu_ref : Outport  Port=4
  eta_ref_end : Outport  Port=5
  nu_ref_end : Outport  Port=6
  WPi_out : Outport  Port=7
  wires:
  eta_ice/1 -> desired unreferenced ship position/1(eta_ice)
  WP/1 -> "End system, after last WP is reached "/1(WP), "Initiation system, try to DP at point some deg out from the WP-start"/1(WP)
  eta_ship/1 -> Velocity reference/2(eta_ship)
  alpha_LOS/1 -> Velocity reference/1(alpha_LOS), desired unreferenced ship position/2(alpha_LOS)
  "Initiation system, try to DP at point some deg out from the WP-start"/1(eta_ref_ship) -> eta_ref_ini/1
  desired unreferenced ship position/1(eta_ref ship) -> eta_ref/1
  Velocity reference/1(nu_ref ship) -> nu_ref/1
  WPi/1 -> WPi_out/1
  "End system, after last WP is reached "/2(nu_ref_end) -> nu_ref_end/1
  "End system, after last WP is reached "/1(eta_ref_end) -> eta_ref_end/1
  alpha_LOS_saved/1 -> "End system, after last WP is reached "/2(alphaLOS_save)
  "Initiation system, try to DP at point some deg out from the WP-start"/2(nu_ref_ship) -> nu_ref_ini/1
  delta_rup/1 -> Velocity reference/3(delta_rup)

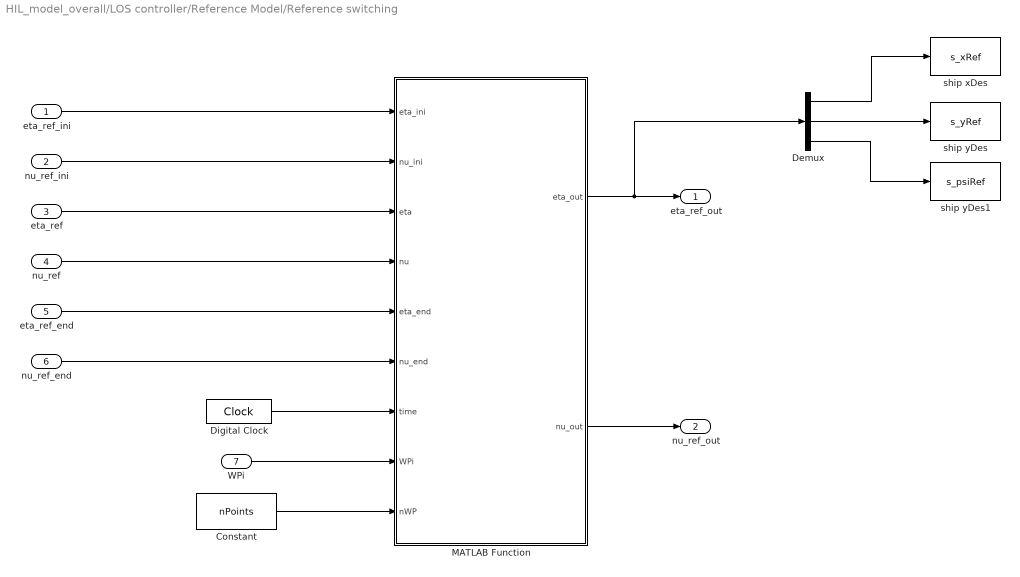
== system HIL_model_overall/LOS controller/Reference Model/Reference switching ==
  eta_ref_ini : Inport
  nu_ref_ini : Inport  Port=2
  eta_ref : Inport  Port=3
  nu_ref : Inport  Port=4
  eta_ref_end : Inport  Port=5
  nu_ref_end : Inport  Port=6
  WPi : Inport  Port=7
  Constant : Constant  Value=nPoints
  Demux : Demux  Outputs=3
  Digital Clock : DigitalClock  SampleTime=0.1
  MATLAB Function : MATLAB Function  TreatAsAtomicUnit=on
  ship xDes : ToWorkspace  VariableName=s_xRef  SaveFormat=Timeseries  SampleTime=-1
  ship yDes : ToWorkspace  VariableName=s_yRef  SaveFormat=Timeseries  SampleTime=-1
  ship yDes1 : ToWorkspace  VariableName=s_psiRef  SaveFormat=Timeseries  SampleTime=-1
  eta_ref_out : Outport
  nu_ref_out : Outport  Port=2
  wires:
  eta_ref_ini/1 -> MATLAB Function/1(eta_ini)
  nu_ref_ini/1 -> MATLAB Function/2(nu_ini)
  eta_ref/1 -> MATLAB Function/3(eta)
  nu_ref/1 -> MATLAB Function/4(nu)
  Digital Clock/1 -> MATLAB Function/7(time)
  MATLAB Function/1(eta_out) -> Demux/1, eta_ref_out/1
  MATLAB Function/2(nu_out) -> nu_ref_out/1
  eta_ref_end/1 -> MATLAB Function/5(eta_end)
  nu_ref_end/1 -> MATLAB Function/6(nu_end)
  WPi/1 -> MATLAB Function/8(WPi)
  Constant/1 -> MATLAB Function/9(nWP)
  Demux/1 -> ship xDes/1
  Demux/2 -> ship yDes/1
  Demux/3 -> ship yDes1/1

== system HIL_model_overall/Nonlinear Passive Observer Towing vessel/estimation/b_s hat ==
  eta_s error : Inport
  Integrator2 : Integrator  InitialCondition=[0; 0; 0]
  K3 : Gain  Gain=K3_obs  Multiplication=Matrix(K*u)
  Sum2 : Sum  Inputs=+-
  T bias : Gain  Gain=inv(T_bias)  Multiplication=Matrix(K*u)
  b_s hat : Outport
  wires:
  T bias/1 -> Sum2/2
  Integrator2/1 -> T bias/1, b_s hat/1  "b_s hat"
  Sum2/1 -> Integrator2/1
  K3/1 -> Sum2/1
  eta_s error/1 -> K3/1

== system HIL_model_overall/Nonlinear Passive Observer Towing vessel/estimation/eta_s hat ==
  eta_s error : Inport
  Rs : Inport  Port=2
  nu_s hat : Inport  Port=3
  Integrator : Integrator  InitialCondition=Pship
  K2 : Gain  Gain=K2_obs  Multiplication=Matrix(K*u)
  Product : Product  Multiplication=Matrix(*)
  Sum : Sum
  eta_s hat : Outport
  wires:
  nu_s hat/1 -> Product/2
  Sum/1 -> Integrator/1
  Rs/1 -> Product/1
  Product/1 -> Sum/2
  eta_s error/1 -> K2/1
  Integrator/1 -> eta_s hat/1
  K2/1 -> Sum/1

== system HIL_model_overall/Nonlinear Passive Observer Towing vessel/estimation/nu_s hat ==
  Rst : Inport
  Tau : Inport  Port=2
  eta_s error : Inport  Port=3
  b_s hat : Inport  Port=4
  D : Gain  Gain=Ds  Multiplication=Matrix(K*u)
  Integrator1 : Integrator  InitialCondition=[0; 0; 0]
  K4 : Constant  Value=K4_obs  VectorParams1D=off
  M-1 : Gain  Gain=inv(Ms_tot)  Multiplication=Matrix(K*u)
  Product1 : Product  Multiplication=Matrix(*)
  Product2 : Product  Inputs=***  Multiplication=Matrix(*)
  Sum1 : Sum  Inputs=-+++
  nu_s hat : Outport
  wires:
  b_s hat/1 -> Product1/2
  Rst/1 -> Product2/1, Product1/1
  Product1/1 -> Sum1/3
  M-1/1 -> Integrator1/1
  Integrator1/1 -> D/1, nu_s hat/1
  Tau/1 -> Sum1/2
  K4/1 -> Product2/2
  D/1 -> Sum1/1
  Product2/1 -> Sum1/4
  Sum1/1 -> M-1/1
  eta_s error/1 -> Product2/3

== system HIL_model_overall/HIL Model - CS Enterprise I->towline->iceberg/Ship - Iceberg - Current Model/Current model/Subsystem ==
  nu_c : Inport
  r : Inport  Port=2
  Constant : Constant  Value=0
  Demux : Demux  Outputs=3
  Gain : Gain  Gain=-1
  Product : Product
  Product1 : Product
  Terminator : Terminator
  Vector Concatenate : Concatenate  NumInputs=3  Mode=Multidimensional array
  nu_c_dot : Outport
  wires:
  Gain/1 -> Product1/2
  Demux/1 -> Gain/1
  Demux/2 -> Product/2
  r/1 -> Product/1, Product1/1
  Constant/1 -> Vector Concatenate/3
  Product1/1 -> Vector Concatenate/2
  Product/1 -> Vector Concatenate/1
  Vector Concatenate/1 -> nu_c_dot/1
  Demux/3 -> Terminator/1
  nu_c/1 -> Demux/1

== system HIL_model_overall/LOS controller/Reference Model/Reference models/End system, after last WP is reached  ==
  WP : Inport
  alphaLOS_save : Inport  Port=2
  Constant : Constant  Value=TowLineLength + shipL_d(1)
  MATLAB Function : MATLAB Function  TreatAsAtomicUnit=on
  eta_ref_end : Outport
  nu_ref_end : Outport  Port=2
  wires:
  MATLAB Function/1(eta_ref_end) -> eta_ref_end/1
  WP/1 -> MATLAB Function/2(WP)
  Constant/1 -> MATLAB Function/1(L)
  MATLAB Function/2(nu_ref_end) -> nu_ref_end/1
  alphaLOS_save/1 -> MATLAB Function/3(alphaLOS_saved)

== system HIL_model_overall/LOS controller/Reference Model/Reference models/Initiation system, try to DP at point some deg out from the WP-start ==
  WP : Inport
  Constant : Constant  Value=TowLineLength
  Constant1 : Constant  Value=shipL_d(1)
  Constant2 : Constant  Value=Offset_direction
  Constant3 : Constant  Value=0
  MATLAB Function : MATLAB Function  TreatAsAtomicUnit=on
  Mux : Mux  Inputs=3
  eta_ref_ship : Outport
  nu_ref_ship : Outport  Port=2
  wires:
  MATLAB Function/1(eta_ref) -> eta_ref_ship/1
  WP/1 -> MATLAB Function/1(WP)
  Constant/1 -> MATLAB Function/2(L_rope)
  Constant1/1 -> MATLAB Function/3(L_fast)
  Constant2/1 -> MATLAB Function/4(Offset_direction)
  Constant3/1 -> Mux/3, Mux/2, Mux/1
  Mux/1 -> nu_ref_ship/1

== system HIL_model_overall/LOS controller/Reference Model/Reference models/Velocity reference ==
  alpha_LOS : Inport
  eta_ship : Inport  Port=2
  delta_rup : Inport  Port=3
  Clock : Clock
  Constant : Constant  Value=u_ref
  Constant1 : Constant  Value=0
  Constant4 : Constant  Value=ruptureNear
  Constant5 : Constant  Value=ruptureLimitRef
  MATLAB Function : MATLAB Function  TreatAsAtomicUnit=on
  MATLAB Function1 : MATLAB Function  TreatAsAtomicUnit=on
  Mux : Mux  Inputs=3
  To Workspace : ToWorkspace  VariableName=delta_pen  SaveFormat=Timeseries  SampleTime=-1
  To Workspace1 : ToWorkspace  VariableName=Uref  SaveFormat=Timeseries  SampleTime=-1
  delta_T penalty : Subsystem
  nu_ref ship : Outport
  wires:
  Mux/1 -> nu_ref ship/1
  eta_ship/1 -> MATLAB Function/2(eta_ship)
  alpha_LOS/1 -> MATLAB Function/3(alpha_LOS)
  MATLAB Function/2(sway) -> Mux/2
  MATLAB Function/1(surge) -> Mux/1
  Constant1/1 -> Mux/3
  delta_T penalty/1(U_ref) -> MATLAB Function/1(U), To Workspace1/1
  Constant5/1 -> delta_T penalty/3(delta_lim)
  Constant4/1 -> delta_T penalty/4(delta_care)
  delta_rup/1 -> delta_T penalty/2(delta_T)
  delta_T penalty/2(delta_penalty out) -> To Workspace/1
  MATLAB Function1/1(U_ref) -> delta_T penalty/1(U in)
  Constant/1 -> MATLAB Function1/1(U_in)
  Clock/1 -> MATLAB Function1/2(t)

== system HIL_model_overall/LOS controller/Reference Model/Reference models/desired unreferenced ship position ==
  eta_ice : Inport
  alpha_LOS : Inport  Port=2
  Demux : Demux  Outputs=2
  L_fastening to geo center : Constant  Value=shipL_d(1)
  Ltau : Constant  Value=TowLineLength
  Memory : Memory
  Mux : Mux  Inputs=2
  Mux1 : Mux  Inputs=3
  Product : Product
  Sum : Sum
  Sum1 : Sum
  Trigonometric Function : Trigonometry
  Trigonometric Function1 : Trigonometry  Operator=cos
  "pi -> inf" : MATLAB Function  TreatAsAtomicUnit=on
  eta_ref ship : Outport
  wires:
  alpha_LOS/1 -> Trigonometric Function/1, "pi -> inf"/1(alpha_pi), Trigonometric Function1/1
  eta_ice/1 -> Sum/1
  Ltau/1 -> Sum1/1
  L_fastening to geo center/1 -> Sum1/2
  Trigonometric Function1/1 -> Mux/1
  Trigonometric Function/1 -> Mux/2
  Sum1/1 -> Product/1
  Mux/1 -> Product/2
  Product/1 -> Sum/2
  Sum/1 -> Demux/1
  Mux1/1 -> eta_ref ship/1
  Demux/1 -> Mux1/1
  Demux/2 -> Mux1/2
  "pi -> inf"/1(alpha_inf) -> Memory/1, Mux1/3
  Memory/1 -> "pi -> inf"/2(accumulation)

== system HIL_model_overall/LOS controller/Reference Model/Reference models/Velocity reference/delta_T penalty ==
  U in : Inport
  delta_T : Inport  Port=2
  delta_lim : Inport  Port=3
  delta_care : Inport  Port=4
  Change limiter : MATLAB Function  TreatAsAtomicUnit=on
  Constant : Constant
  Constant2 : Constant  Value=0
  MATLAB Function : MATLAB Function  TreatAsAtomicUnit=on
  Memory : Memory  X0=100  InheritSampleTime=on
  MinMax : MinMax  Inputs=2
  MinMax1 : MinMax  Function=max  Inputs=2
  Product1 : Product
  Sum : Sum  Inputs=|+-
  U_ref : Outport
  delta_penalty out : Outport  Port=2
  wires:
  delta_T/1 -> MATLAB Function/1(deltaT)
  Constant/1 -> MinMax/1, Sum/1
  Product1/1 -> U_ref/1
  U in/1 -> Product1/1
  MinMax/1 -> Sum/2
  Constant2/1 -> MinMax1/1
  MinMax1/1 -> MinMax/2
  MATLAB Function/1(out) -> MinMax1/2
  delta_care/1 -> MATLAB Function/3(delta_care)
  delta_lim/1 -> MATLAB Function/2(delta_lim)
  Change limiter/1(newPen) -> Product1/2, delta_penalty out/1, Memory/1
  Memory/1 -> Change limiter/2(prevPen)
  Sum/1 -> Change limiter/1(pen)

== matlab function HIL_model_overall/HIL Model - CS Enterprise I->towline->iceberg/Ship - Iceberg - Current Model/MC Lab Signal Fault ==
  data: error output; err_percent input; eta_s output; eta_s_in input; eta_i_in input; error_previous input; eta_s_previous input; eta_i_previous input; eta_i output
function [error, eta_s, eta_i] = fcn(err_percent, eta_s_in, eta_i_in, error_previous, eta_s_previous, eta_i_previous)
%#codegen


% Random number generator 0-100
num = 100*rand;

if error_previous == 1
    err_percent = 95;
end

% Check if the num is below the error percentage
if num < err_percent
    error = 1;
    eta_s = eta_s_previous;
    eta_i = eta_i_previous;
else
    error = 0;
    eta_s = eta_s_in;
    eta_i = eta_i_in;
end

== matlab function HIL_model_overall/HIL Model - CS Enterprise I->towline->iceberg/Ship - Iceberg - Current Model/Ship model/R(psi)1 ==
  data: psi input; R output
function R = fcn(psi)

c = cos(psi);
s = sin(psi);

R = [c -s 0;
     s c 0;
     0 0 1];

== matlab function HIL_model_overall/delta index/Mean ==
  data: counter output; theCount input; N input; Mean output; StandardDev output; input input; saved_in input; saved_out output
function [counter, Mean, StandardDev, saved_out] = fcn(theCount, N, input, saved_in)
%#codegen

meanSum = 0;
varSum = 0;

N = round(N);

startval = 2;
Ndiv = N;
if theCount < N
    startval = N + 1 - theCount;
    Ndiv = theCount;
end

% Bump all saved instances up
saved_out = saved_in;
for i=startval:N
    saved_out(i-1) = saved_in(i);
    meanSum = meanSum + saved_in(i);
end
saved_out(N) = input;
meanSum = meanSum + input;

Mean = (1/Ndiv)*meanSum;


% Calculate variance sum
for i=startval-1:N
    varSum = (saved_out(i) - Mean)^2;
end

variance = (1/Ndiv)*varSum;
StandardDev = sqrt(variance);

counter = theCount + 1;

== matlab function HIL_model_overall/HIL Model - CS Enterprise I->towline->iceberg/Tension estimator/Tension estimate ==
  data: eta_s_in input; Tension output; eta_i_in input; TowLineParameters input; T output; disconnected input
function [Tension, T] = fcn(eta_s_in,eta_i_in,TowLineParameters, disconnected)
%#codegen

if length(eta_s_in) > 1
    eta_s = eta_s_in;
else
    eta_s = [0; 0; 0];
end
if length(eta_i_in) > 1
    eta_i = eta_i_in;
else
    eta_i = [0; 0];
end

if disconnected == 0

    d = TowLineParameters(1);
    Tlength = TowLineParameters(2);
    K_tow = TowLineParameters(3);

    x_s = eta_s(1);
    y_s = eta_s(2);
    psi_s = eta_s(3);

    x_i = eta_i(1);
    y_i = eta_i(2);

    % Find rope fastening position in cartesian
    x_r = x_s - d*cos(psi_s);
    y_r = y_s - d*sin(psi_s);

    % Find towline fastening distance and angle
    dist = sqrt( (x_r - x_i)^2 + (y_r - y_i)^2 );
    angle = atan2(y_r-y_i, x_r-x_i);

    % Check if longer than rope length, because only rope stretching tension gives force
    T = 0;
    if dist >= Tlength

        deltaL = dist-Tlength;
        T = K_tow*deltaL;

    end

    % Make Xtow and Ytow
    Xtow = T*cos(angle);
    Ytow = T*sin(angle);

    Tension = [Xtow; Ytow];

else
    
    T = 0;
    Tension = [0; 0];
    
end

== matlab function HIL_model_overall/Failure modes/MATLAB Function ==
  data: deltaIndex input; disconnect output; limits input; preDisconnect input; theTime input
function disconnect = fcn(deltaIndex, limits, preDisconnect, theTime)
%#codegen

disconnect = preDisconnect;

if preDisconnect == 0 && theTime > 0

    deltaOverturn = deltaIndex(3);
    deltaRupture = deltaIndex(1);
    deltaSlippage = deltaIndex(2);
    
    overturn = limits(1);
    rupture = limits(2);
    slippage = limits(3);
    
    if deltaOverturn < overturn

        theTime
        disp('Iceberg has overturned, towline is disconnected.');
        disconnect = 1;
        
    elseif deltaRupture < rupture
        
        theTime
        disp('Towline has ruptured, and is disconnected.');
        disconnect = 1;
        
    elseif deltaSlippage < slippage
        
        theTime
        disp('Towline has slipped, and is disconnected.');
        disconnect = 1;
        
    end
    
end
